simulink model "SV_Modulation"  (R2018a)
settings: Solver=VariableStepAuto  StartTime=0.0  StopTime=.3  FixedStep=.000001  MaxStep=.00001  RelTol=1e-3
libraries: simulink x1
settings Model: Creator=Hossam  LastModifiedBy=Hossam

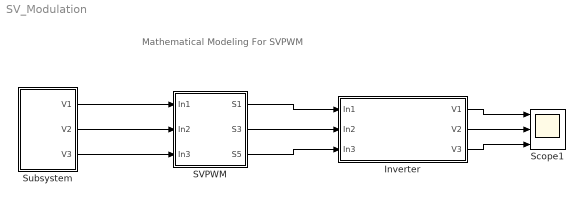
== system SV_Modulation ==
  note: Mathematical Modeling For SVPWM
  Inverter : Subsystem  TreatAsAtomicUnit=on
  SVPWM : Subsystem  TreatAsAtomicUnit=on
  Scope1 : Scope  NumInputPorts=3
  Subsystem : Subsystem  mask{Vp=197.600}
      mask prompts: Vp "Vpeak"
  wires:
  SVPWM/3(S5) -> Inverter/3(In3)
  SVPWM/1(S1) -> Inverter/1(In1)
  SVPWM/2(S3) -> Inverter/2(In2)
  Inverter/1(V1) -> Scope1/1
  Inverter/2(V2) -> Scope1/2
  Inverter/3(V3) -> Scope1/3
  Subsystem/1(V1) -> SVPWM/1(In1)
  Subsystem/2(V2) -> SVPWM/2(In2)
  Subsystem/3(V3) -> SVPWM/3(In3)

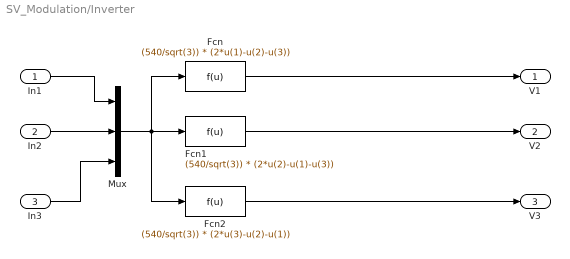
== system SV_Modulation/Inverter ==
  In1 : Inport  OutDataTypeStr=double
  In2 : Inport  Port=2  OutDataTypeStr=double
  In3 : Inport  Port=3  OutDataTypeStr=double
  Fcn : Fcn  Expr=(540/sqrt(3)) * (2*u(1)-u(2)-u(3))
  Fcn1 : Fcn  Expr=(540/sqrt(3)) * (2*u(2)-u(1)-u(3))
  Fcn2 : Fcn  Expr=(540/sqrt(3)) * (2*u(3)-u(2)-u(1))
  Mux : Mux  Inputs=3
  V1 : Outport
  V2 : Outport  Port=2
  V3 : Outport  Port=3
  wires:
  Mux/1 -> Fcn2/1, Fcn/1, Fcn1/1
  In1/1 -> Mux/1
  In2/1 -> Mux/2
  In3/1 -> Mux/3
  Fcn/1 -> V1/1
  Fcn2/1 -> V3/1
  Fcn1/1 -> V2/1

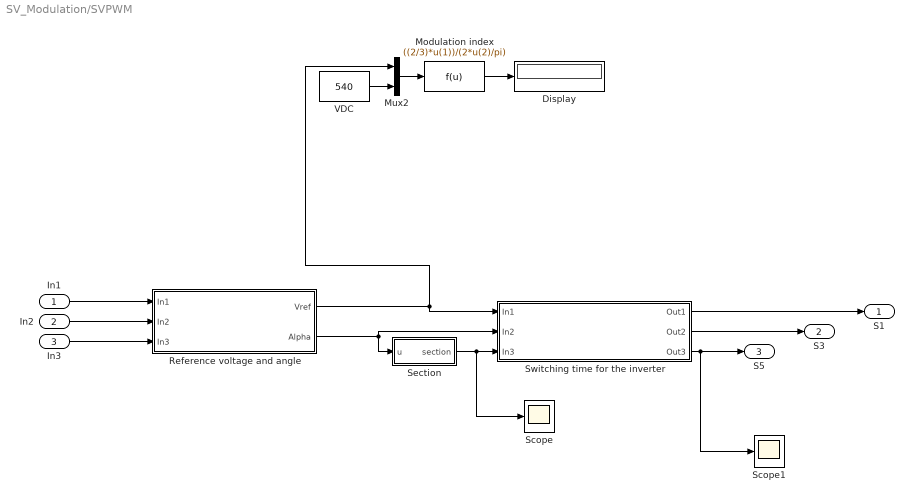
== system SV_Modulation/SVPWM ==
  In1 : Inport
  In2 : Inport  Port=2
  In3 : Inport  Port=3
  Display : Display
  Modulation index : Fcn  Expr=((2/3)*u(1))/(2*u(2)/pi)
  Mux2 : Mux  Inputs=2
  Reference voltage and angle : Subsystem
  Scope : Scope
  Scope1 : Scope
  "Section " : MATLAB Function  TreatAsAtomicUnit=on
  Switching time for the inverter : Subsystem
  VDC : Constant  Value=540
  S1 : Outport
  S3 : Outport  Port=2
  S5 : Outport  Port=3
  wires:
  Mux2/1 -> Modulation index/1
  VDC/1 -> Mux2/2
  Modulation index/1 -> Display/1
  "Section "/1(section) -> Scope/1, Switching time for the inverter/3(In3)
  Switching time for the inverter/1(Out1) -> S1/1
  Switching time for the inverter/2(Out2) -> S3/1
  Switching time for the inverter/3(Out3) -> Scope1/1, S5/1
  Reference voltage and angle/2(Alpha) -> Switching time for the inverter/2(In2), "Section "/1(u)
  Reference voltage and angle/1(Vref) -> Switching time for the inverter/1(In1), Mux2/1
  In1/1 -> Reference voltage and angle/1(In1)
  In2/1 -> Reference voltage and angle/2(In2)
  In3/1 -> Reference voltage and angle/3(In3)

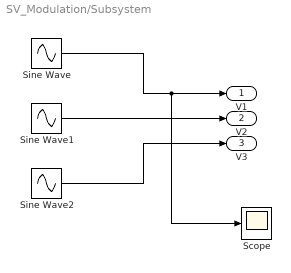
== system SV_Modulation/Subsystem ==
  Scope : Scope
  Sine Wave : Sin  Amplitude=Vp*sqrt(2)  Frequency=2*pi*50  SampleTime=0
  Sine Wave1 : Sin  Amplitude=Vp*sqrt(2)  Frequency=2*pi*50  Phase=-2*pi/3  SampleTime=0
  Sine Wave2 : Sin  Amplitude=Vp*sqrt(2)  Frequency=2*pi*50  Phase=2*pi/3  SampleTime=0
  V1 : Outport
  V2 : Outport  Port=2
  V3 : Outport  Port=3
  wires:
  Sine Wave/1 -> Scope/1, V1/1
  Sine Wave1/1 -> V2/1
  Sine Wave2/1 -> V3/1

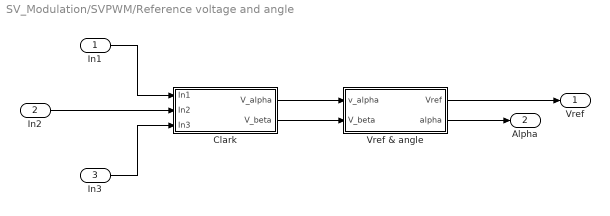
== system SV_Modulation/SVPWM/Reference voltage and angle ==
  In1 : Inport
  In2 : Inport  Port=2
  In3 : Inport  Port=3
  Clark : Subsystem
  Vref & angle : Subsystem
  Vref : Outport
  Alpha : Outport  Port=2
  wires:
  Clark/1(V_alpha) -> Vref & angle/1(v_alpha)
  In3/1 -> Clark/3(In3)
  Vref & angle/2(alpha) -> Alpha/1
  Clark/2(V_beta) -> Vref & angle/2(V_beta)
  In2/1 -> Clark/2(In2)
  Vref & angle/1(Vref) -> Vref/1
  In1/1 -> Clark/1(In1)

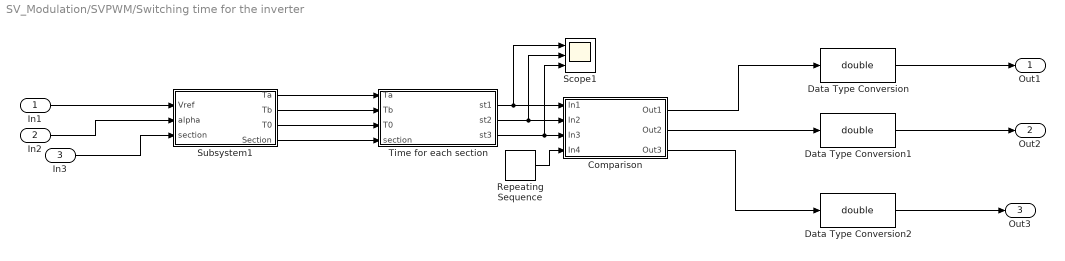
== system SV_Modulation/SVPWM/Switching time for the inverter ==
  In1 : Inport
  In2 : Inport  Port=2
  In3 : Inport  Port=3
  Comparison : Subsystem
  Data Type Conversion : DataTypeConversion  OutDataTypeStr=double
  Data Type Conversion1 : DataTypeConversion  OutDataTypeStr=double
  Data Type Conversion2 : DataTypeConversion  OutDataTypeStr=double
  Repeating Sequence : simulink/Sources/Repeating Sequence  rep_seq_t=[0 1/5000]  rep_seq_y=[-1 1]
  Scope1 : Scope  NumInputPorts=3
  Subsystem1 : Subsystem
  Time for each section : MATLAB Function  TreatAsAtomicUnit=on
  Out1 : Outport
  Out2 : Outport  Port=2
  Out3 : Outport  Port=3
  wires:
  Subsystem1/2(Tb) -> Time for each section/2(Tb)
  Time for each section/1(st1) -> Scope1/1, Comparison/1(In1)
  Subsystem1/3(T0) -> Time for each section/3(T0)
  Subsystem1/4(Section) -> Time for each section/4(section)
  Subsystem1/1(Ta) -> Time for each section/1(Ta)
  Comparison/2(Out2) -> Data Type Conversion1/1
  Time for each section/2(st2) -> Scope1/2, Comparison/2(In2)
  Time for each section/3(st3) -> Scope1/3, Comparison/3(In3)
  In3/1 -> Subsystem1/3(section)
  In1/1 -> Subsystem1/1(Vref)
  In2/1 -> Subsystem1/2(alpha)
  Comparison/3(Out3) -> Data Type Conversion2/1
  Comparison/1(Out1) -> Data Type Conversion/1
  Repeating Sequence/1 -> Comparison/4(In4)
  Data Type Conversion/1 -> Out1/1
  Data Type Conversion2/1 -> Out3/1
  Data Type Conversion1/1 -> Out2/1

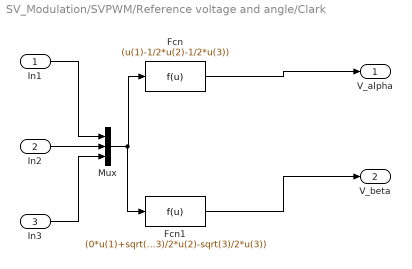
== system SV_Modulation/SVPWM/Reference voltage and angle/Clark ==
  In1 : Inport
  In2 : Inport  Port=2
  In3 : Inport  Port=3
  Fcn : Fcn  Expr=(u(1)-1/2*u(2)-1/2*u(3))
  Fcn1 : Fcn  Expr=(0*u(1)+sqrt(3)/2*u(2)-sqrt(3)/2*u(3))
  Mux : Mux  Inputs=3
  V_alpha : Outport
  V_beta : Outport  Port=2
  wires:
  Fcn1/1 -> V_beta/1
  Fcn/1 -> V_alpha/1
  Mux/1 -> Fcn1/1, Fcn/1
  In1/1 -> Mux/1
  In2/1 -> Mux/2
  In3/1 -> Mux/3

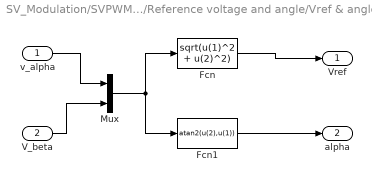
== system SV_Modulation/SVPWM/Reference voltage and angle/Vref & angle ==
  v_alpha : Inport
  V_beta : Inport  Port=2
  Fcn : Fcn  Expr=sqrt(u(1)^2 + u(2)^2)
  Fcn1 : Fcn  Expr=atan2(u(2),u(1))
  Mux : Mux  Inputs=2
  Vref : Outport
  alpha : Outport  Port=2
  wires:
  Fcn/1 -> Vref/1
  Fcn1/1 -> alpha/1
  v_alpha/1 -> Mux/1
  V_beta/1 -> Mux/2
  Mux/1 -> Fcn1/1, Fcn/1

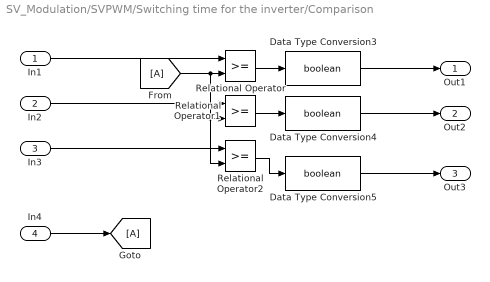
== system SV_Modulation/SVPWM/Switching time for the inverter/Comparison ==
  In1 : Inport
  In2 : Inport  Port=2
  In3 : Inport  Port=3
  In4 : Inport  Port=4
  Data Type Conversion3 : DataTypeConversion  OutDataTypeStr=boolean
  Data Type Conversion4 : DataTypeConversion  OutDataTypeStr=boolean
  Data Type Conversion5 : DataTypeConversion  OutDataTypeStr=boolean
  Relational Operator : RelationalOperator  OutDataTypeStr=boolean  RndMeth=Simplest
  Relational Operator1 : RelationalOperator  OutDataTypeStr=boolean  RndMeth=Simplest
  Relational Operator2 : RelationalOperator  OutDataTypeStr=boolean  RndMeth=Simplest
  Out1 : Outport
  Out2 : Outport  Port=2
  Out3 : Outport  Port=3
  wires:
  In1/1 -> Relational Operator/1
  In2/1 -> Relational Operator1/1
  In3/1 -> Relational Operator2/1
  In4/1 -> [A]
  [A] -> Relational Operator2/2, Relational Operator1/2, Relational Operator/2
  Data Type Conversion3/1 -> Out1/1
  Data Type Conversion5/1 -> Out3/1
  Data Type Conversion4/1 -> Out2/1
  Relational Operator/1 -> Data Type Conversion3/1
  Relational Operator1/1 -> Data Type Conversion4/1
  Relational Operator2/1 -> Data Type Conversion5/1

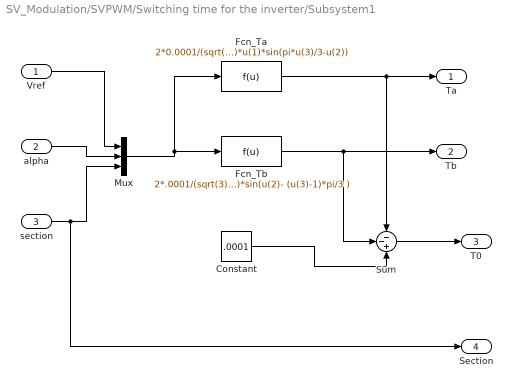
== system SV_Modulation/SVPWM/Switching time for the inverter/Subsystem1 ==
  Vref : Inport
  alpha : Inport  Port=2
  section : Inport  Port=3
  Constant : Constant  Value=.0001
  Fcn_Ta : Fcn  Expr=2*0.0001/(sqrt(3)*380)*u(1)*sin(pi*u(3)/3-u(2))
  Fcn_Tb : Fcn  Expr=2*.0001/(sqrt(3)*380)*u(1)*sin(u(2)- (u(3)-1)*pi/3 )
  Mux : Mux  Inputs=3
  Sum : Sum  Inputs=--+
  Ta : Outport
  Tb : Outport  Port=2
  T0 : Outport  Port=3
  Section : Outport  Port=4
  wires:
  Fcn_Ta/1 -> Sum/1, Ta/1
  Fcn_Tb/1 -> Sum/2, Tb/1
  Constant/1 -> Sum/3
  Sum/1 -> T0/1
  Mux/1 -> Fcn_Tb/1, Fcn_Ta/1
  Vref/1 -> Mux/1
  alpha/1 -> Mux/2
  section/1 -> Section/1, Mux/3

== matlab function SV_Modulation/SVPWM/Switching time for the inverter/Time for each section ==
  data: Ta input; st1 output; Tb input; T0 input; section input; st2 output; st3 output
function [st1,st2,st3]= fcn(Ta,Tb,T0,section)
Tperiod=.0001;
if section==1
    st1= Tperiod - (T0/2);
    st2= (T0/2)+ Tb ;
    st3= (T0/2) ;
elseif section==2
    st1= (T0/2)+ Ta ;
    st2= Tperiod - (T0/2);
    st3= (T0/2) ;
elseif section==3
    st1= (T0/2) ;
    st2= Tperiod - (T0/2);
    st3= (T0/2)+ Tb ;
elseif section==4
    st1= (T0/2) ;
    st2=  (T0/2)+ Ta ;
    st3= Tperiod - (T0/2);
elseif section==5
    st1= (T0/2)+ Tb ;
    st2=  (T0/2) ;
    st3= Tperiod - (T0/2);
else
    st1= Tperiod - (T0/2);
    st2=  (T0/2) ;
    st3= (T0/2)+ Ta;
end
end

== matlab function SV_Modulation/SVPWM/Section  ==
  data: u input; section output
function section = fcn(u)
 u= 360/(2*pi)*u ; 
if (u>=0)&&(u<60)
    section=1;
elseif(u>=60)&&(u<120)
    section=2;
elseif (u>=120)&&(u<180)
    section=3;
elseif (u>=-180)&&(u<-120)
    section=4;
elseif (u>=-120)&&(u<-60)
    section=5;
elseif (u>=-60) && (u<0)
    section=6;
else 
    section=0;
end
end
